simulink model "Sixphase_PMSM_VSD_Robj"  (R2023b)
settings: Solver=ode23t  StartTime=0.0  StopTime=0.5  RelTol=1e-4  EnableMultiTasking=on
InitFcn:
  | Ts=1e-6;
undefined symbols (not defined in the file): DiscIntNeverNeededParam
libraries: spsVoltageMeasurementLib x4, powerlib_extras x3, spsUniversalBridgeLib x2, spsDCVoltageSourceLib x1, spspowerguiLib x1
settings Model: Creator=y  LastModifiedBy=Guoguo
settings SolverCC: AlgebraicLoopSolver=TrustRegion
settings DataIOCC: LimitDataPoints=on  SaveFormat=Array  SignalLoggingSaveFormat=ModelDataLogs  ReturnWorkspaceOutputs=off
settings OptimizationCC: ExpressionDepthLimit=2147483647  InitFltsAndDblsToZero=on  LifeSpan=inf
settings DebuggingCC: SaveWithParameterizedLinksMsg=none  UnderspecifiedInitializationDetection=Classic  MergeDetectMultiDrivingBlocksExec=none  SignalResolutionControl=TryResolveAllWithWarning  SolverPrmCheckMsg=warning  MultiTaskDSMMsg=warning  MultiTaskCondExecSysMsg=none  FcnCallInpInsideContextMsg=warning  UnconnectedInputMsg=warning  UnconnectedOutputMsg=warning  UnconnectedLineMsg=warning  StateNameClashWarn=warning  SFUnexpectedBacktrackingDiag=warning  SFNoUnconditionalDefaultTransitionDiag=warning  SFExecutionAtInitializationDiag=none  ArithmeticOperatorsInVariantConditions=warning
settings HardwareCC: ProdBitPerPointer=32  ProdBitPerSizeT=32  ProdBitPerPtrDiffT=32  ProdLargestAtomicFloat=None  ProdIntDivRoundTo=Undefined  ProdEndianess=Unspecified  ProdWordSize=32  ProdHWDeviceType=32-bit Generic
settings ModelReferenceCC: EnableRefExpFcnMdlSchedulingChecks=on  PropagateSignalLabelsOutOfModel=off
settings SFSimCC: SimUseLocalCustomCode=off  CustomCodeUndefinedFunction=UseInterfaceOnly
settings RTWCC: RTWUseLocalCustomCode=off  DLArmComputeVersion=19.05
settings CodeAppCC: StateflowObjectComments=on
settings GRTTargetCC: TargetFcnLib=ansi_tfl_tmw.mat  TargetLangStandard=C89/C90 (ANSI)  CombineOutputUpdateFcns=off  GRTInterface=on
settings ConfigComp: CovMetricSettings=dw  CovSaveCumulativeToWorkspaceVar=on  CovSaveSingleToWorkspaceVar=on  CovExternalEMLEnable=off  CovSFcnEnable=off
settings SimscapeCC: SimscapeNormalizeSystem=off

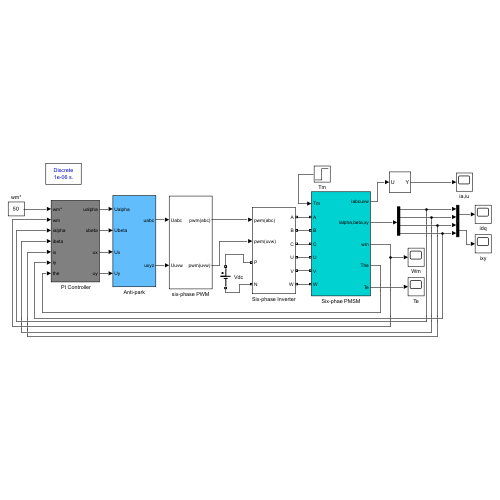
[thumbnail: Simulink's stored preview of the top-level diagram]
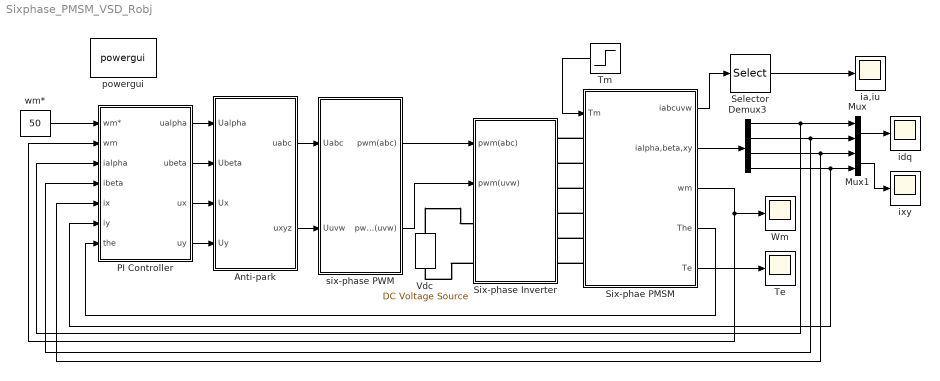
== system Sixphase_PMSM_VSD_Robj ==
  " PI Controller" : Subsystem
  Anti-park : Subsystem
  Demux3 : Demux
  Mux : Mux  Inputs=2
  Mux1 : Mux  Inputs=2
  Selector : Selector  InputPortWidth=6  IndexOptions=Index vector (dialog)  Indices=[1 4]  OutputSizes=1
  Six-phae PMSM : Subsystem  mask{R=1.4, Ld=0.008, Lq=0.008, Lz=0.0017, Flux=0.68, J=0.015, F=0, p=3}
      mask prompts: R "R(ohm)"; Ld "Ld(H)"; Lq "Lq(H)"; Lz "Lz(H)"; Flux "Flux(Wb)"; J "J(kg.m^2)"; F "F(N.m.s)"
  Six-phase Inverter : Subsystem
  Te : Scope
  Tm : Step  Time=0.2  After=50  SampleTime=0
  Vdc : spsDCVoltageSourceLib/DC Voltage Source  Amplitude=400  Measurements=None
  Wm : Scope
  ia,iu : Scope
  idq : Scope
  ixy : Scope
  powergui : spspowerguiLib/powergui  Priority=1  SimulationMode=Discrete  SampleTime=1e-6  frequency=60  Iterations=50  frequencyindice=0  Pbase=100e6  ErrMax=1e-4  UnitsV=kV  UnitsW=MW  buscounter=0  FunctionMessages=off  echomessages=off  EnableUseOfTLC=off  CurrentSourceSwitches=on  DisableSnubberDevices=off  DisableRonSwitches=off  DisableVfSwitches=off  DisplayEquations=off  AutomaticDiscreteSolvers=off  SolverType=Tustin/Backward Euler (TBE)  Interpol=off  ExternalGateDelay=off  methode=off  Ts=100  x0status=blocks  SPID=off  SwTol=0  HookPort=off  NonlinearTolerance=1e-4  nMaxIteration=100  ContinueOnMaxIteration=off  RestoreLinks=warning  ResistiveCurrentMeasurement=off  Frange=[0:2:500]  Ylog=off  Xlog=on  ShowGrid=off  save=off  variable=ZData  structure=iau  ZoomFFT=off  StartTime=0.4  cycles=2  DisplayStyle=1  fundamental=25  FreqAxis=off  MaxFrequency=1000  frequencyindicesteady=1  RmsSteady=1  display=off
  six-phase PWM : Subsystem
  wm* : Constant  Value=50
  wires:
  Six-phae PMSM/4(The) -> " PI Controller"/7(the)
  wm*/1 -> " PI Controller"/1(wm*)
  Six-phae PMSM/2(ialpha,beta,xy) -> Demux3/1
  Six-phae PMSM/5(Te) -> Te/1
  " PI Controller"/1(ualpha) -> Anti-park/1(Ualpha)
  " PI Controller"/2(ubeta) -> Anti-park/2(Ubeta)
  " PI Controller"/3(ux) -> Anti-park/3(Ux)
  " PI Controller"/4(uy) -> Anti-park/4(Uy)
  Demux3/1 -> Mux/1, " PI Controller"/3(ialpha)
  Demux3/2 -> Mux/2, " PI Controller"/4(ibeta)
  Demux3/3 -> " PI Controller"/5(ix), Mux1/1
  Demux3/4 -> " PI Controller"/6(iy), Mux1/2
  Tm/1 -> Six-phae PMSM/1(Tm)
  Anti-park/1(uabc) -> six-phase PWM/1(Uabc)
  Anti-park/2(uxyz) -> six-phase PWM/2(Uuvw)
  six-phase PWM/1(pwm(abc)) -> Six-phase Inverter/1(pwm(abc))
  six-phase PWM/2(pwm(uvw)) -> Six-phase Inverter/2(pwm(uvw))
  Six-phae PMSM/3(wm) -> Wm/1, " PI Controller"/2(wm)
  Mux/1 -> idq/1
  Mux1/1 -> ixy/1
  Selector/1 -> ia,iu/1
  Six-phae PMSM/1(iabcuvw) -> Selector/1
  connections:
  Six-phae PMSM/LConn1 -- Six-phase Inverter/RConn1
  Six-phae PMSM/LConn2 -- Six-phase Inverter/RConn2
  Six-phae PMSM/LConn3 -- Six-phase Inverter/RConn3
  Six-phae PMSM/LConn4 -- Six-phase Inverter/RConn4
  Six-phae PMSM/LConn5 -- Six-phase Inverter/RConn5
  Six-phae PMSM/LConn6 -- Six-phase Inverter/RConn6
  Vdc/RConn1 -- Six-phase Inverter/LConn1
  Six-phase Inverter/LConn2 -- Vdc/LConn1

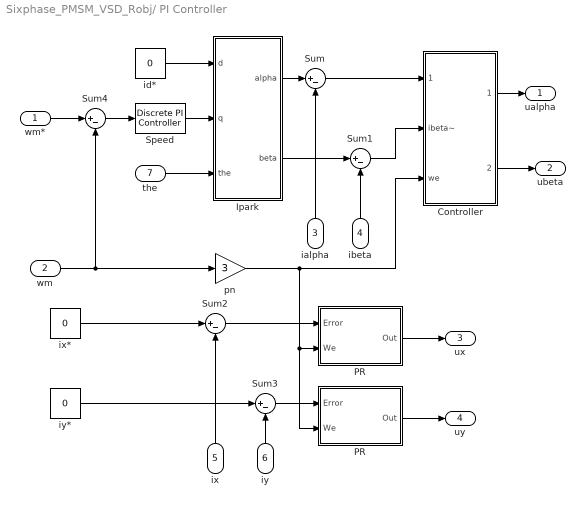
== system Sixphase_PMSM_VSD_Robj/ PI Controller ==
  wm* : Inport
  wm : Inport  Port=2
  ialpha : Inport  Port=3
  ibeta : Inport  Port=4
  ix : Inport  Port=5
  iy : Inport  Port=6
  the : Inport  Port=7
  Controller : Subsystem  AncestorBlock=|  DialogController=POWERSYS.PowerSysDialog  mask(Discrete PI Controller){Kp=0.008*1200, Ki=1.4*1200, Par_Limits=[100 -100], Init=0, Ts=Ts}
      | powerlib_extras/Discrete 
      | Control Blocks/Discrete
      | PI Controller
      mask prompts: Kp "Proportional gain (Kp):"; Ki "Integral gain (Ki):"; Par_Limits "Output limits: [ Upper   Lower ]"; Init "Output initial value:"; Ts "Sample time:"
      mask help: This block implements a discrete PI controller.
      mask init:
      | UpperLimit=Par_Limits(1);
      | LowerLimit=Par_Limits(2);
      | power_initmask();
      mask Help: This block is part of a subset of blocks in the Extras library that does not have documentation associated with it, other than the block mask description.
  Ipark : Subsystem
  PR : Subsystem  AncestorBlock=|  DialogController=POWERSYS.PowerSysDialog  mask(Discrete PI Controller){Kp=0.0017*1200, wc=20, ki=100, Par_Limits=[300/sqrt(3) -300/sqrt(3)], Init=0, Ts=Ts}
      | powerlib_extras/Discrete 
      | Control Blocks/Discrete
      | PI Controller
      mask prompts: Kp "Proportional gain (Kp):"; wc "Cut-off frequency(wc)"; ki "PR integral gain (ki)"; Par_Limits "Output limits: [ Upper   Lower ]"; Init "Output initial value:"; Ts "Sample time:"
      mask help: This block implements a discrete PI controller.
      mask init:
      | UpperLimit=Par_Limits(1);
      | LowerLimit=Par_Limits(2);
      | power_initmask();
      mask Help: This block is part of a subset of blocks in the Extras library that does not have documentation associated with it, other than the block mask description.
  "PR " : Subsystem  AncestorBlock=|  DialogController=POWERSYS.PowerSysDialog  mask(Discrete PI Controller){Kp=0.0017*1200, wc=20, ki=100, Par_Limits=[300/sqrt(3) -300/sqrt(3)], Init=0, Ts=Ts}
      | powerlib_extras/Discrete 
      | Control Blocks/Discrete
      | PI Controller
      mask prompts: Kp "Proportional gain (Kp):"; wc "Cut-off frequency(wc)"; ki "PR integral gain (ki)"; Par_Limits "Output limits: [ Upper   Lower ]"; Init "Output initial value:"; Ts "Sample time:"
      mask help: This block implements a discrete PI controller.
      mask init:
      | UpperLimit=Par_Limits(1);
      | LowerLimit=Par_Limits(2);
      | power_initmask();
      mask Help: This block is part of a subset of blocks in the Extras library that does not have documentation associated with it, other than the block mask description.
  Speed : powerlib_extras/Discrete  Control Blocks/Discrete PI Controller  Kp=1  Ki=80  Par_Limits=[25 -25]  Init=0  Ts=Ts
  Sum{,1..4} (5 alike) : Sum  Inputs=|+-
  id* : Constant  Value=0
  ix* : Constant  Value=0
  iy* : Constant  Value=0
  pn : Gain  Gain=3
  ualpha : Outport
  ubeta : Outport  Port=2
  ux : Outport  Port=3
  uy : Outport  Port=4
  wires:
  Sum3/1 -> "PR "/1(Error)
  Sum2/1 -> PR/1(Error)
  Sum1/1 -> Controller/2(ibeta~)
  Sum/1 -> Controller/1(ialpha~)
  Sum4/1 -> Speed/1
  ix/1 -> Sum2/2
  iy/1 -> Sum3/2
  Controller/1(Valpha*) -> ualpha/1
  Controller/2(Vbeta*) -> ubeta/1
  ix*/1 -> Sum2/1
  iy*/1 -> Sum3/1
  PR/1(Out) -> ux/1
  "PR "/1(Out) -> uy/1
  Ipark/1(alpha) -> Sum/1
  id*/1 -> Ipark/1(d)
  Speed/1 -> Ipark/2(q)
  Ipark/2(beta) -> Sum1/1
  the/1 -> Ipark/3(the)
  ialpha/1 -> Sum/2
  ibeta/1 -> Sum1/2
  wm/1 -> pn/1, Sum4/2
  wm*/1 -> Sum4/1
  pn/1 -> "PR "/2(We), PR/2(We), Controller/3(we)

== system Sixphase_PMSM_VSD_Robj/Anti-park ==
  Ualpha : Inport
  Ubeta : Inport  Port=2
  Ux : Inport  Port=3
  Uy : Inport  Port=4
  Demux : Demux  Outputs=2
  Gain : Gain  Gain=1/200
  IClarke-6 : Subsystem
  uabc : Outport
  uxyz : Outport  Port=2
  wires:
  IClarke-6/1(ABCUVW) -> Gain/1
  Ualpha/1 -> IClarke-6/1(alpha)
  Ubeta/1 -> IClarke-6/2(beta)
  Ux/1 -> IClarke-6/3(x)
  Uy/1 -> IClarke-6/4(y)
  Gain/1 -> Demux/1
  Demux/1 -> uabc/1
  Demux/2 -> uxyz/1

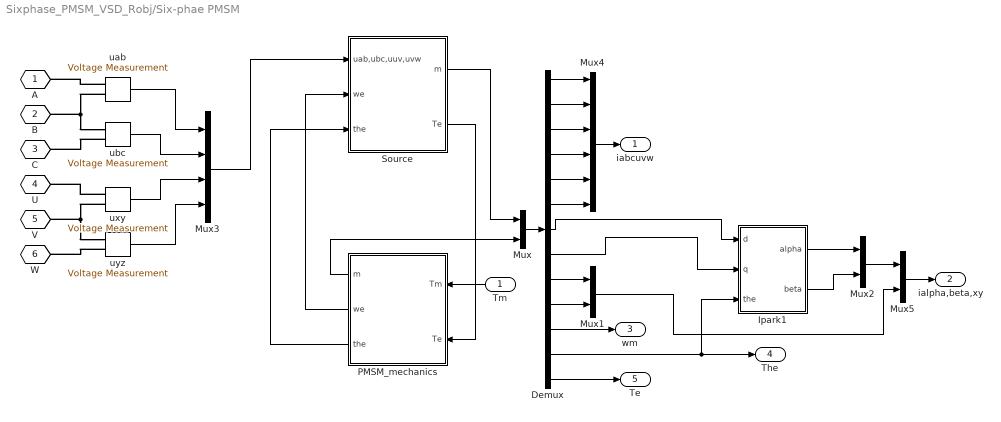
== system Sixphase_PMSM_VSD_Robj/Six-phae PMSM ==
  Tm : Inport
  Demux : Demux  Outputs=13
  Ipark1 : Subsystem
  Mux{,1..2,5} (4 alike) : Mux  Inputs=2
  Mux3 : Mux
  Mux4 : Mux  Inputs=6
  PMSM_mechanics : Subsystem
  Source : Subsystem
  uab : spsVoltageMeasurementLib/Voltage Measurement  PhasorSimulation=off  OutputType=Complex  PSBequivalent=0
  ubc : spsVoltageMeasurementLib/Voltage Measurement  PhasorSimulation=off  OutputType=Complex  PSBequivalent=0
  uxy : spsVoltageMeasurementLib/Voltage Measurement  PhasorSimulation=off  OutputType=Complex  PSBequivalent=0
  uyz : spsVoltageMeasurementLib/Voltage Measurement  PhasorSimulation=off  OutputType=Complex  PSBequivalent=0
  A : PMIOPort  Tag=PMCPort  Side=Left
  B : PMIOPort  Tag=PMCPort  Port=2  Side=Left
  C : PMIOPort  Tag=PMCPort  Port=3  Side=Left
  U : PMIOPort  Tag=PMCPort  Port=4  Side=Left
  V : PMIOPort  Tag=PMCPort  Port=5  Side=Left
  W : PMIOPort  Tag=PMCPort  Port=6  Side=Left
  iabcuvw : Outport
  ialpha,beta,xy : Outport  Port=2
  wm : Outport  Port=3
  The : Outport  Port=4
  Te : Outport  Port=5
  wires:
  Tm/1 -> PMSM_mechanics/1(Tm)
  Source/2(Te) -> PMSM_mechanics/2(Te)
  PMSM_mechanics/2(we) -> Source/2(we)
  PMSM_mechanics/3(the) -> Source/3(the)
  PMSM_mechanics/1(m) -> Mux/2
  Source/1(m) -> Mux/1
  Mux3/1 -> Source/1(uab,ubc,uuv,uvw)
  Mux/1 -> Demux/1
  Mux4/1 -> iabcuvw/1
  Mux5/1 -> ialpha,beta,xy/1
  Demux/12 -> Ipark1/3(the), The/1
  Demux/13 -> Te/1
  uab/1 -> Mux3/1
  ubc/1 -> Mux3/2
  uxy/1 -> Mux3/3
  uyz/1 -> Mux3/4
  Demux/5 -> Mux4/5
  Demux/2 -> Mux4/2
  Demux/3 -> Mux4/3
  Demux/6 -> Mux4/6
  Demux/4 -> Mux4/4
  Demux/1 -> Mux4/1
  Demux/7 -> Ipark1/1(d)
  Demux/8 -> Ipark1/2(q)
  Demux/9 -> Mux1/1
  Demux/10 -> Mux1/2
  Demux/11 -> wm/1
  Ipark1/1(alpha) -> Mux2/1
  Ipark1/2(beta) -> Mux2/2
  Mux2/1 -> Mux5/1
  Mux1/1 -> Mux5/2
  connections:
  uab/LConn1 -- A/RConn1
  uab/LConn2 -- B/RConn1 -- ubc/LConn1
  ubc/LConn2 -- C/RConn1
  uxy/LConn1 -- U/RConn1
  uxy/LConn2 -- V/RConn1 -- uyz/LConn1
  uyz/LConn2 -- W/RConn1

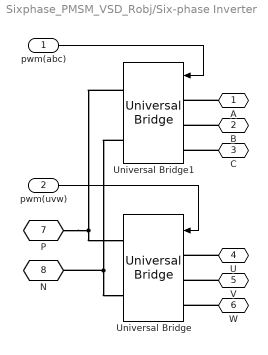
== system Sixphase_PMSM_VSD_Robj/Six-phase Inverter ==
  pwm(abc) : Inport
  pwm(uvw) : Inport  Port=2
  Universal Bridge : spsUniversalBridgeLib/Universal Bridge  Arms=3  SnubberResistance=1e5  SnubberCapacitance=inf  Device=IGBT / Diodes  Ron=1e-3  Lon=0  ForwardVoltages="[  0  0  ]"  ForwardVoltage=0  GTOparameters=[ 10e-6 , 20e-6 ]  IGBTparameters=[ 1e-6 , 2e-6 ]  Measurements=None  Measurements_2=None  converterType=Rectifier
  Universal Bridge1 : spsUniversalBridgeLib/Universal Bridge  Arms=3  SnubberResistance=1e5  SnubberCapacitance=inf  Device=IGBT / Diodes  Ron=1e-3  Lon=0  ForwardVoltages="[  0  0  ]"  ForwardVoltage=0  GTOparameters=[ 10e-6 , 20e-6 ]  IGBTparameters=[ 1e-6 , 2e-6 ]  Measurements=None  Measurements_2=None  converterType=Rectifier
  A : PMIOPort  Side=Right
  B : PMIOPort  Port=2  Side=Right
  C : PMIOPort  Port=3  Side=Right
  U : PMIOPort  Port=4  Side=Right
  V : PMIOPort  Port=5  Side=Right
  W : PMIOPort  Port=6  Side=Right
  P : PMIOPort  Port=7  Side=Left
  N : PMIOPort  Port=8  Side=Left
  wires:
  pwm(abc)/1 -> Universal Bridge1/1
  pwm(uvw)/1 -> Universal Bridge/1
  connections:
  A/RConn1 -- Universal Bridge1/LConn1
  C/RConn1 -- Universal Bridge1/LConn3
  W/RConn1 -- Universal Bridge/LConn3
  B/RConn1 -- Universal Bridge1/LConn2
  U/RConn1 -- Universal Bridge/LConn1
  V/RConn1 -- Universal Bridge/LConn2
  Universal Bridge1/RConn1 -- P/RConn1 -- Universal Bridge/RConn1
  Universal Bridge1/RConn2 -- N/RConn1 -- Universal Bridge/RConn2

== system Sixphase_PMSM_VSD_Robj/six-phase PWM ==
  Uabc : Inport
  Uuvw : Inport  Port=2
  Discrete PWM Generator : powerlib_extras/Discrete  Control Blocks/Discrete PWM Generator  GeneratorMode="3-arm  bridge (6 pulses)"  Fc=10000  Ts=1e-6  Internal=off  mIndex=0.4  Freq=60  Phase=0
  Discrete PWM Generator1 : powerlib_extras/Discrete  Control Blocks/Discrete PWM Generator  GeneratorMode="3-arm  bridge (6 pulses)"  Fc=10000  Ts=1e-6  Internal=off  mIndex=0.4  Freq=60  Phase=0
  pwm(abc) : Outport
  pwm(uvw) : Outport  Port=2
  wires:
  Uabc/1 -> Discrete PWM Generator/1
  Discrete PWM Generator1/1 -> pwm(uvw)/1
  Uuvw/1 -> Discrete PWM Generator1/1
  Discrete PWM Generator/1 -> pwm(abc)/1

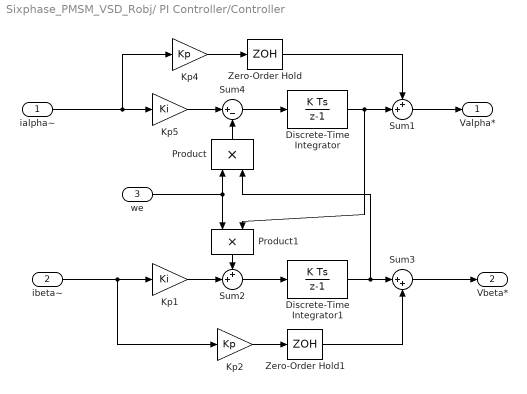
== system Sixphase_PMSM_VSD_Robj/ PI Controller/Controller ==
  ialpha~ : Inport  SampleTime=Ts
  ibeta~ : Inport  Port=2  SampleTime=Ts
  we : Inport  Port=3  SampleTime=Ts
  Discrete-Time Integrator : DiscreteIntegrator  InitialCondition=Init  SampleTime=Ts  UpperSaturationLimit=UpperLimit  LowerSaturationLimit=LowerLimit  ICPrevOutput=DiscIntNeverNeededParam  ICPrevScaledInput=DiscIntNeverNeededParam
  Discrete-Time Integrator1 : DiscreteIntegrator  InitialCondition=Init  SampleTime=Ts  UpperSaturationLimit=UpperLimit  LowerSaturationLimit=LowerLimit  ICPrevOutput=DiscIntNeverNeededParam  ICPrevScaledInput=DiscIntNeverNeededParam
  Kp1 : Gain  Gain=Ki  SaturateOnIntegerOverflow=on  SampleTime=Ts  OutDataTypeStr=Inherit: Same as input  ParamDataTypeStr=Inherit: Same as input
  Kp2 : Gain  Gain=Kp  SaturateOnIntegerOverflow=on  SampleTime=Ts  OutDataTypeStr=Inherit: Same as input  ParamDataTypeStr=Inherit: Same as input
  Kp4 : Gain  Gain=Kp  SaturateOnIntegerOverflow=on  SampleTime=Ts  OutDataTypeStr=Inherit: Same as input  ParamDataTypeStr=Inherit: Same as input
  Kp5 : Gain  Gain=Ki  SaturateOnIntegerOverflow=on  SampleTime=Ts  OutDataTypeStr=Inherit: Same as input  ParamDataTypeStr=Inherit: Same as input
  Product : Product
  Product1 : Product
  Sum1 : Sum  Inputs=++|
  Sum2 : Sum  Inputs=++|
  Sum3 : Sum  Inputs=|++
  Sum4 : Sum  Inputs=|+-
  Zero-Order Hold : ZeroOrderHold  SampleTime=Ts
  Zero-Order Hold1 : ZeroOrderHold  SampleTime=Ts
  Valpha* : Outport  SampleTime=Ts  InitialOutput=0
  Vbeta* : Outport  Port=2  SampleTime=Ts  InitialOutput=0
  wires:
  ialpha~/1 -> Kp4/1, Kp5/1
  Kp4/1 -> Zero-Order Hold/1
  Sum1/1 -> Valpha*/1
  Zero-Order Hold/1 -> Sum1/1
  Kp5/1 -> Sum4/1
  Sum4/1 -> Discrete-Time Integrator/1
  Product/1 -> Sum4/2
  we/1 -> Product1/1, Product/1
  Sum2/1 -> Discrete-Time Integrator1/1
  Kp1/1 -> Sum2/2
  Kp2/1 -> Zero-Order Hold1/1
  ibeta~/1 -> Kp2/1, Kp1/1
  Zero-Order Hold1/1 -> Sum3/2
  Discrete-Time Integrator1/1 -> Product/2, Sum3/1
  Product1/1 -> Sum2/1
  Discrete-Time Integrator/1 -> Product1/2, Sum1/2
  Sum3/1 -> Vbeta*/1

== system Sixphase_PMSM_VSD_Robj/ PI Controller/Ipark ==
  d : Inport
  q : Inport  Port=2
  the : Inport  Port=3
  Fcn : Fcn  Expr=u[1]*u[4]-u[2]*u[3]
  Fcn1 : Fcn  Expr=u[1]*u[3]+u[2]*u[4]
  Mux : Mux
  cos : Trigonometry  Operator=cos
  sin : Trigonometry
  alpha : Outport
  beta : Outport  Port=2
  wires:
  d/1 -> Mux/1
  q/1 -> Mux/2
  Mux/1 -> Fcn1/1, Fcn/1
  sin/1 -> Mux/3
  cos/1 -> Mux/4
  the/1 -> sin/1, cos/1
  Fcn/1 -> alpha/1
  Fcn1/1 -> beta/1

== system Sixphase_PMSM_VSD_Robj/ PI Controller/PR ==
  note: Discrete PID Controller
  note: Pierre Giroux, Gilbert Sybille
      | Power System Simulation Laboratory
      | IREQ, Hydro-Quebc
  Error : Inport  SampleTime=Ts
  We : Inport  Port=2  SampleTime=Ts
  Kp4 : Gain  Gain=Kp  SaturateOnIntegerOverflow=on  SampleTime=Ts  OutDataTypeStr=Inherit: Same as input  ParamDataTypeStr=Inherit: Same as input
  PR : Subsystem
  Sum6 : Sum  InputSameDT=on  SaturateOnIntegerOverflow=on  SampleTime=Ts  OutDataTypeStr=Inherit: Same as first input
  Zero-Order Hold : ZeroOrderHold  SampleTime=Ts
  Out : Outport  SampleTime=Ts  InitialOutput=0
  wires:
  PR/1(Out) -> Sum6/2
  We/1 -> PR/2(we)
  Zero-Order Hold/1 -> Sum6/1
  Sum6/1 -> Out/1
  Kp4/1 -> Zero-Order Hold/1
  Error/1 -> PR/1(error), Kp4/1

== system Sixphase_PMSM_VSD_Robj/ PI Controller/PR  ==
  note: Pierre Giroux, Gilbert Sybille
      | Power System Simulation Laboratory
      | IREQ, Hydro-Quebc
  note: Discrete PID Controller
  Error : Inport  SampleTime=Ts
  We : Inport  Port=2  SampleTime=Ts
  Kp4 : Gain  Gain=Kp  SaturateOnIntegerOverflow=on  SampleTime=Ts  OutDataTypeStr=Inherit: Same as input  ParamDataTypeStr=Inherit: Same as input
  PR : Subsystem
  Sum6 : Sum  InputSameDT=on  SaturateOnIntegerOverflow=on  SampleTime=Ts  OutDataTypeStr=Inherit: Same as first input
  Zero-Order Hold : ZeroOrderHold  SampleTime=Ts
  Out : Outport  SampleTime=Ts  InitialOutput=0
  wires:
  Error/1 -> Kp4/1, PR/1(error)
  Kp4/1 -> Zero-Order Hold/1
  Sum6/1 -> Out/1
  Zero-Order Hold/1 -> Sum6/1
  We/1 -> PR/2(we)
  PR/1(Out) -> Sum6/2

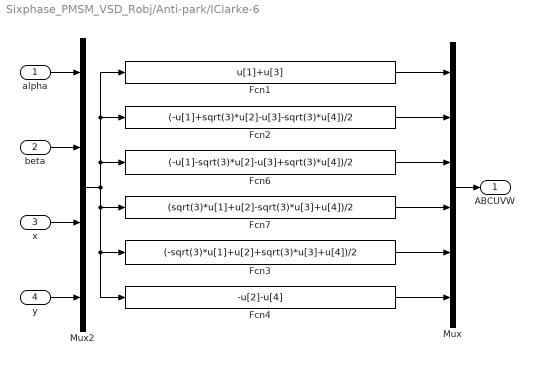
== system Sixphase_PMSM_VSD_Robj/Anti-park/IClarke-6 ==
  alpha : Inport
  beta : Inport  Port=2
  x : Inport  Port=3
  y : Inport  Port=4
  Fcn1 : Fcn  Expr=u[1]+u[3]
  Fcn2 : Fcn  Expr=(-u[1]+sqrt(3)*u[2]-u[3]-sqrt(3)*u[4])/2
  Fcn3 : Fcn  Expr=(-sqrt(3)*u[1]+u[2]+sqrt(3)*u[3]+u[4])/2
  Fcn4 : Fcn  Expr=-u[2]-u[4]
  Fcn6 : Fcn  Expr=(-u[1]-sqrt(3)*u[2]-u[3]+sqrt(3)*u[4])/2
  Fcn7 : Fcn  Expr=(sqrt(3)*u[1]+u[2]-sqrt(3)*u[3]+u[4])/2
  Mux : Mux  Inputs=6
  Mux2 : Mux
  ABCUVW : Outport
  wires:
  alpha/1 -> Mux2/1
  beta/1 -> Mux2/2
  x/1 -> Mux2/3
  y/1 -> Mux2/4
  Mux2/1 -> Fcn7/1, Fcn3/1, Fcn4/1, Fcn1/1, Fcn2/1, Fcn6/1
  Fcn1/1 -> Mux/1
  Fcn2/1 -> Mux/2
  Fcn6/1 -> Mux/3
  Fcn7/1 -> Mux/4
  Fcn3/1 -> Mux/5
  Fcn4/1 -> Mux/6
  Mux/1 -> ABCUVW/1

== system Sixphase_PMSM_VSD_Robj/Six-phae PMSM/Ipark1 ==
  d : Inport
  q : Inport  Port=2
  the : Inport  Port=3
  Fcn : Fcn  Expr=u[1]*u[4]-u[2]*u[3]
  Fcn1 : Fcn  Expr=u[1]*u[3]+u[2]*u[4]
  Mux : Mux
  cos : Trigonometry  Operator=cos
  sin : Trigonometry
  alpha : Outport
  beta : Outport  Port=2
  wires:
  Fcn1/1 -> beta/1
  Fcn/1 -> alpha/1
  the/1 -> cos/1, sin/1
  cos/1 -> Mux/4
  sin/1 -> Mux/3
  Mux/1 -> Fcn/1, Fcn1/1
  q/1 -> Mux/2
  d/1 -> Mux/1

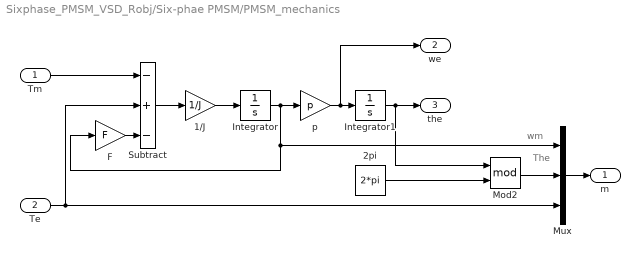
== system Sixphase_PMSM_VSD_Robj/Six-phae PMSM/PMSM_mechanics ==
  note: The
  note: wm
  Tm : Inport
  Te : Inport  Port=2
  1/J : Gain  Gain=1/J
  2pi : Constant  Value=2*pi
  F : Gain  Gain=F
  Integrator : Integrator
  Integrator1 : Integrator
  Mod2 : Math  Operator=mod  SignedPower=on
  Mux : Mux  Inputs=3
  Subtract : Sum  Inputs=-+-
  p : Gain  Gain=p
  m : Outport
  we : Outport  Port=2
  the : Outport  Port=3
  wires:
  Tm/1 -> Subtract/1
  Te/1 -> Subtract/2, Mux/3
  Subtract/1 -> 1/J/1
  1/J/1 -> Integrator/1
  Integrator/1 -> p/1, F/1, Mux/1
  F/1 -> Subtract/3
  p/1 -> Integrator1/1, we/1
  Integrator1/1 -> the/1, Mod2/1
  Mux/1 -> m/1
  Mod2/1 -> Mux/2
  2pi/1 -> Mod2/2

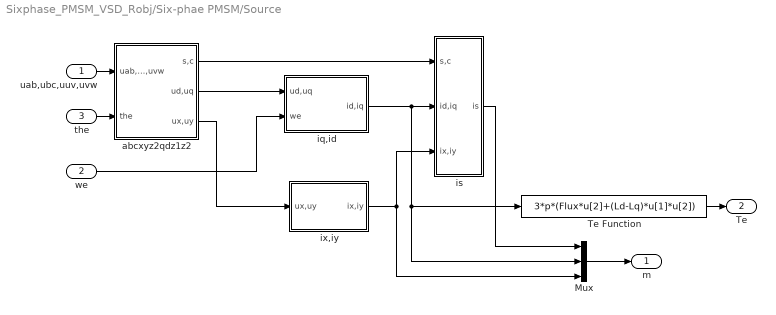
== system Sixphase_PMSM_VSD_Robj/Six-phae PMSM/Source ==
  uab,ubc,uuv,uvw : Inport
  we : Inport  Port=2
  the : Inport  Port=3
  Mux : Mux  Inputs=3
  Te Function : Fcn  Expr=3*p*(Flux*u[2]+(Ld-Lq)*u[1]*u[2])
  abcxyz2qdz1z2 : Subsystem
  iq,id : Subsystem
  is : Subsystem
  ix,iy : Subsystem
  m : Outport
  Te : Outport  Port=2
  wires:
  uab,ubc,uuv,uvw/1 -> abcxyz2qdz1z2/1(uab,ubc,uuv,uvw)
  the/1 -> abcxyz2qdz1z2/2(the)
  abcxyz2qdz1z2/2(ud,uq) -> iq,id/1(ud,uq)
  we/1 -> iq,id/2(we)
  abcxyz2qdz1z2/1(s,c) -> is/1(s,c)
  iq,id/1(id,iq) -> is/2(id,iq), Mux/2, Te Function/1
  Te Function/1 -> Te/1
  abcxyz2qdz1z2/3(ux,uy) -> ix,iy/1(ux,uy)
  ix,iy/1(ix,iy) -> is/3(ix,iy), Mux/3
  Mux/1 -> m/1
  is/1(is) -> Mux/1

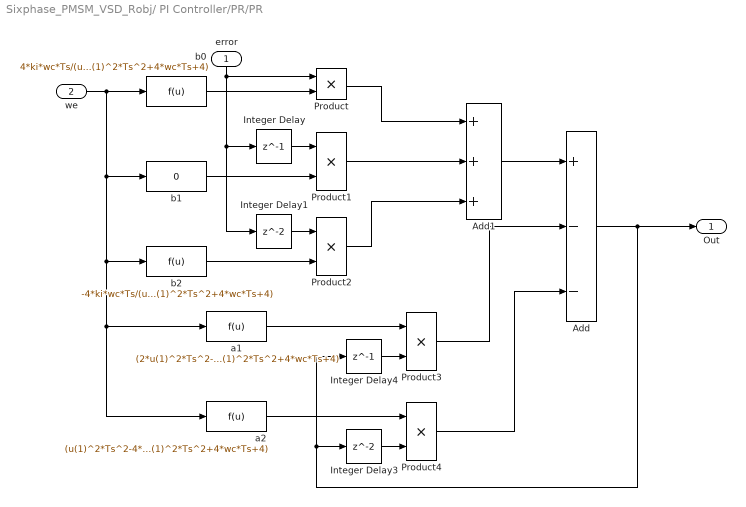
== system Sixphase_PMSM_VSD_Robj/ PI Controller/PR/PR ==
  error : Inport
  we : Inport  Port=2
  Add : Sum  Inputs=+--
  Add1 : Sum  Inputs=+++
  Integer Delay : Delay  DelayLength=1  SampleTime=Ts
  Integer Delay1 : Delay  SampleTime=Ts
  Integer Delay3 : Delay
  Integer Delay4 : Delay  DelayLength=1  SampleTime=Ts
  Product{,1..4} (5 alike) : Product  RndMeth=Zero
  a1 : Fcn  Expr=(2*u(1)^2*Ts^2-8)/(u(1)^2*Ts^2+4*wc*Ts+4)  SampleTime=Ts
  a2 : Fcn  Expr=(u(1)^2*Ts^2-4*wc*Ts+4)/(u(1)^2*Ts^2+4*wc*Ts+4)  SampleTime=Ts
  b0 : Fcn  Expr=4*ki*wc*Ts/(u(1)^2*Ts^2+4*wc*Ts+4)
  b1 : Fcn  Expr=0
  b2 : Fcn  Expr=-4*ki*wc*Ts/(u(1)^2*Ts^2+4*wc*Ts+4)
  Out : Outport
  wires:
  we/1 -> b0/1, b1/1, b2/1, a1/1, a2/1
  b0/1 -> Product/2
  b1/1 -> Product1/2
  Integer Delay/1 -> Product1/1
  Integer Delay1/1 -> Product2/1
  b2/1 -> Product2/2
  Product/1 -> Add1/1
  Product1/1 -> Add1/2
  Product2/1 -> Add1/3
  Add/1 -> Out/1, Integer Delay4/1, Integer Delay3/1
  a1/1 -> Product3/1
  a2/1 -> Product4/1
  Integer Delay3/1 -> Product4/2
  Integer Delay4/1 -> Product3/2
  Add1/1 -> Add/1
  Product3/1 -> Add/2
  Product4/1 -> Add/3
  error/1 -> Product/1, Integer Delay/1, Integer Delay1/1

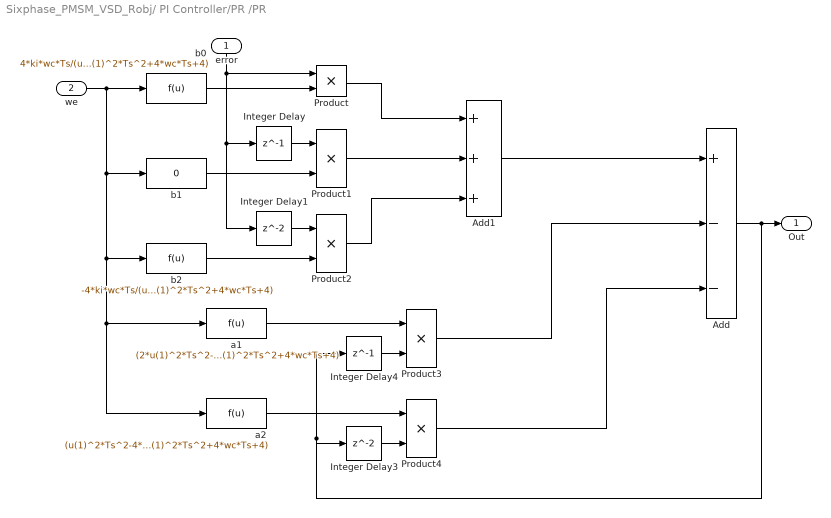
== system Sixphase_PMSM_VSD_Robj/ PI Controller/PR /PR ==
  error : Inport
  we : Inport  Port=2
  Add : Sum  Inputs=+--
  Add1 : Sum  Inputs=+++
  Integer Delay : Delay  DelayLength=1  SampleTime=Ts
  Integer Delay1 : Delay  SampleTime=Ts
  Integer Delay3 : Delay
  Integer Delay4 : Delay  DelayLength=1  SampleTime=Ts
  Product{,1..4} (5 alike) : Product  RndMeth=Zero
  a1 : Fcn  Expr=(2*u(1)^2*Ts^2-8)/(u(1)^2*Ts^2+4*wc*Ts+4)  SampleTime=Ts
  a2 : Fcn  Expr=(u(1)^2*Ts^2-4*wc*Ts+4)/(u(1)^2*Ts^2+4*wc*Ts+4)  SampleTime=Ts
  b0 : Fcn  Expr=4*ki*wc*Ts/(u(1)^2*Ts^2+4*wc*Ts+4)
  b1 : Fcn  Expr=0
  b2 : Fcn  Expr=-4*ki*wc*Ts/(u(1)^2*Ts^2+4*wc*Ts+4)
  Out : Outport
  wires:
  error/1 -> Integer Delay1/1, Integer Delay/1, Product/1
  Product4/1 -> Add/3
  Product3/1 -> Add/2
  Add1/1 -> Add/1
  Integer Delay4/1 -> Product3/2
  Integer Delay3/1 -> Product4/2
  a2/1 -> Product4/1
  a1/1 -> Product3/1
  Add/1 -> Out/1, Integer Delay3/1, Integer Delay4/1
  Product2/1 -> Add1/3
  Product1/1 -> Add1/2
  Product/1 -> Add1/1
  b2/1 -> Product2/2
  Integer Delay1/1 -> Product2/1
  Integer Delay/1 -> Product1/1
  b1/1 -> Product1/2
  b0/1 -> Product/2
  we/1 -> a2/1, a1/1, b2/1, b1/1, b0/1

== system Sixphase_PMSM_VSD_Robj/Six-phae PMSM/Source/abcxyz2qdz1z2 ==
  uab,ubc,uuv,uvw : Inport
  the : Inport  Port=2
  Clarke : Subsystem
  Mux2 : Mux  Inputs=2
  PARK : Subsystem
  Trigonometric Function : Trigonometry
  Trigonometric Function1 : Trigonometry  Operator=cos
  s,c : Outport
  ud,uq : Outport  Port=2
  ux,uy : Outport  Port=3
  wires:
  Mux2/1 -> PARK/2(s,c), s,c/1
  the/1 -> Trigonometric Function1/1, Trigonometric Function/1
  PARK/1(ud,uq) -> ud,uq/1
  uab,ubc,uuv,uvw/1 -> Clarke/1(uab,ubc,uuv,uvw)
  Trigonometric Function1/1 -> Mux2/2
  Trigonometric Function/1 -> Mux2/1
  Clarke/1(ualpha,ubeta) -> PARK/1(ualpha,ubeta)
  Clarke/2(ux,uy) -> ux,uy/1

== system Sixphase_PMSM_VSD_Robj/Six-phae PMSM/Source/iq,id ==
  ud,uq : Inport
  we : Inport  Port=2
  Demux : Demux  Outputs=2
  Mux : Mux  Inputs=2
  id : Subsystem
  iq : Subsystem
  id,iq : Outport
  wires:
  ud,uq/1 -> Demux/1
  Mux/1 -> id,iq/1
  Demux/1 -> id/1(ud)
  Demux/2 -> iq/3(uq)
  we/1 -> iq/2(we), id/2(we)
  iq/1(iq) -> id/3(iq), Mux/2
  id/1(id) -> iq/1(id), Mux/1

== system Sixphase_PMSM_VSD_Robj/Six-phae PMSM/Source/is ==
  s,c : Inport
  id,iq : Inport  Port=2
  ix,iy : Inport  Port=3
  IClarke : Subsystem
  IPARK : Subsystem
  is : Outport
  wires:
  s,c/1 -> IPARK/1(s,c)
  id,iq/1 -> IPARK/2(id,iq)
  IPARK/1(ialpha,ibeta) -> IClarke/1(ialpha,ibeta)
  ix,iy/1 -> IClarke/2(ix,iy)
  IClarke/1(iabcuvw) -> is/1

== system Sixphase_PMSM_VSD_Robj/Six-phae PMSM/Source/ix,iy ==
  ux,uy : Inport
  Demux : Demux  Outputs=2
  Mux : Mux  Inputs=2
  ix : Subsystem
  iy : Subsystem
  ix,iy : Outport
  wires:
  Mux/1 -> ix,iy/1
  ux,uy/1 -> Demux/1
  Demux/1 -> ix/1(ux)
  Demux/2 -> iy/1(uy)
  ix/1(ix) -> Mux/1
  iy/1(iy) -> Mux/2

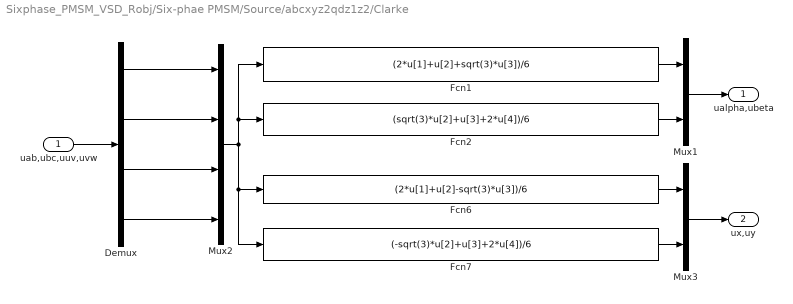
== system Sixphase_PMSM_VSD_Robj/Six-phae PMSM/Source/abcxyz2qdz1z2/Clarke ==
  uab,ubc,uuv,uvw : Inport
  Demux : Demux
  Fcn1 : Fcn  Expr=(2*u[1]+u[2]+sqrt(3)*u[3])/6
  Fcn2 : Fcn  Expr=(sqrt(3)*u[2]+u[3]+2*u[4])/6
  Fcn6 : Fcn  Expr=(2*u[1]+u[2]-sqrt(3)*u[3])/6
  Fcn7 : Fcn  Expr=(-sqrt(3)*u[2]+u[3]+2*u[4])/6
  Mux1 : Mux  Inputs=2
  Mux2 : Mux
  Mux3 : Mux  Inputs=2
  ualpha,ubeta : Outport
  ux,uy : Outport  Port=2
  wires:
  Demux/2 -> Mux2/2
  Demux/3 -> Mux2/3
  Demux/4 -> Mux2/4
  Mux2/1 -> Fcn1/1, Fcn2/1, Fcn6/1, Fcn7/1
  uab,ubc,uuv,uvw/1 -> Demux/1
  Demux/1 -> Mux2/1
  Mux1/1 -> ualpha,ubeta/1
  Fcn1/1 -> Mux1/1
  Fcn2/1 -> Mux1/2
  Fcn6/1 -> Mux3/1
  Fcn7/1 -> Mux3/2
  Mux3/1 -> ux,uy/1

== system Sixphase_PMSM_VSD_Robj/Six-phae PMSM/Source/abcxyz2qdz1z2/PARK ==
  ualpha,ubeta : Inport
  s,c : Inport  Port=2
  Demux : Demux  Outputs=2
  Demux1 : Demux  Outputs=2
  Fcn : Fcn  Expr=u[1]*u[4]+u[2]*u[3]
  Fcn1 : Fcn  Expr=-u[1]*u[3]+u[2]*u[4]
  Mux : Mux
  Mux1 : Mux  Inputs=2
  ud,uq : Outport
  wires:
  Mux/1 -> Fcn/1, Fcn1/1
  s,c/1 -> Demux/1
  ualpha,ubeta/1 -> Demux1/1
  Demux1/1 -> Mux/1
  Demux1/2 -> Mux/2
  Demux/1 -> Mux/3
  Demux/2 -> Mux/4
  Fcn/1 -> Mux1/1
  Fcn1/1 -> Mux1/2
  Mux1/1 -> ud,uq/1

== system Sixphase_PMSM_VSD_Robj/Six-phae PMSM/Source/iq,id/id ==
  ud : Inport
  we : Inport  Port=2
  iq : Inport  Port=3
  1/Ld : Gain  Gain=1/Ld
  Lq/Ld : Gain  Gain=Lq/Ld
  Product : Product  RndMeth=Zero
  R/Ld : Gain  Gain=R/Ld
  Subtract : Sum  Inputs=-++
  d/dt(id) : Integrator
  id : Outport
  wires:
  d/dt(id)/1 -> id/1, R/Ld/1
  Subtract/1 -> d/dt(id)/1
  R/Ld/1 -> Subtract/1
  1/Ld/1 -> Subtract/2
  Lq/Ld/1 -> Subtract/3
  Product/1 -> Lq/Ld/1
  iq/1 -> Product/2
  we/1 -> Product/1
  ud/1 -> 1/Ld/1

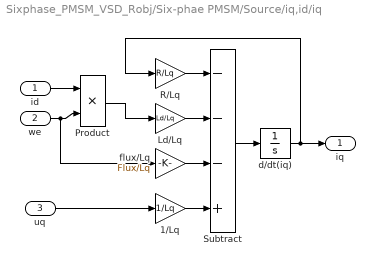
== system Sixphase_PMSM_VSD_Robj/Six-phae PMSM/Source/iq,id/iq ==
  id : Inport
  we : Inport  Port=2
  uq : Inport  Port=3
  1/Lq : Gain  Gain=1/Lq
  Ld/Lq : Gain  Gain=Ld/Lq
  Product : Product  RndMeth=Zero
  R/Lq : Gain  Gain=R/Lq
  Subtract : Sum  Inputs=---+
  d/dt(iq) : Integrator
  flux/Lq : Gain  Gain=Flux/Lq
  iq : Outport
  wires:
  d/dt(iq)/1 -> iq/1, R/Lq/1
  Subtract/1 -> d/dt(iq)/1
  R/Lq/1 -> Subtract/1
  Ld/Lq/1 -> Subtract/2
  flux/Lq/1 -> Subtract/3
  1/Lq/1 -> Subtract/4
  uq/1 -> 1/Lq/1
  we/1 -> Product/2, flux/Lq/1
  id/1 -> Product/1
  Product/1 -> Ld/Lq/1

== system Sixphase_PMSM_VSD_Robj/Six-phae PMSM/Source/is/IClarke ==
  ialpha,ibeta : Inport
  ix,iy : Inport  Port=2
  Fcn1 : Fcn  Expr=u[1]+u[3]
  Fcn2 : Fcn  Expr=-1/2*u[1]+sqrt(3)/2*u[2]-1/2*u[3]-sqrt(3)/2*u[4]
  Fcn3 : Fcn  Expr=-sqrt(3)/2*u[1]+1/2*u[2]+sqrt(3)/2*u[3]+1/2*u[4]
  Fcn4 : Fcn  Expr=-u[2]-u[4]
  Fcn6 : Fcn  Expr=-1/2*u[1]-sqrt(3)/2*u[2]-1/2*u[3]+sqrt(3)/2*u[4]
  Fcn7 : Fcn  Expr=sqrt(3)/2*u[1]+1/2*u[2]-sqrt(3)/2*u[3]+1/2*u[4]
  Mux : Mux  Inputs=6
  Mux2 : Mux  Inputs=2
  iabcuvw : Outport
  wires:
  Mux2/1 -> Fcn1/1, Fcn2/1, Fcn6/1, Fcn7/1, Fcn4/1, Fcn3/1
  Fcn1/1 -> Mux/1
  Fcn2/1 -> Mux/2
  Fcn6/1 -> Mux/3
  Fcn7/1 -> Mux/4
  Fcn3/1 -> Mux/5
  Fcn4/1 -> Mux/6
  Mux/1 -> iabcuvw/1
  ialpha,ibeta/1 -> Mux2/1
  ix,iy/1 -> Mux2/2

== system Sixphase_PMSM_VSD_Robj/Six-phae PMSM/Source/is/IPARK ==
  s,c : Inport
  id,iq : Inport  Port=2
  Demux : Demux  Outputs=2
  Demux1 : Demux  Outputs=2
  Mux : Mux
  Mux1 : Mux  Inputs=2
  ialpha : Fcn  Expr=u[1]*u[4]-u[2]*u[3]
  ibeta : Fcn  Expr=u[1]*u[3]+u[2]*u[4]
  ialpha,ibeta : Outport
  wires:
  Mux/1 -> ibeta/1, ialpha/1
  Demux/2 -> Mux/2
  Demux/1 -> Mux/1
  id,iq/1 -> Demux/1
  Demux1/1 -> Mux/3
  Demux1/2 -> Mux/4
  s,c/1 -> Demux1/1
  ialpha/1 -> Mux1/1
  ibeta/1 -> Mux1/2
  Mux1/1 -> ialpha,ibeta/1

== system Sixphase_PMSM_VSD_Robj/Six-phae PMSM/Source/ix,iy/ix ==
  ux : Inport
  1/Lz : Gain  Gain=1/Lz
  R/Lz : Gain  Gain=R/Lz
  Subtract : Sum  Inputs=-+
  d/dt(ix) : Integrator
  ix : Outport
  wires:
  d/dt(ix)/1 -> ix/1, R/Lz/1
  Subtract/1 -> d/dt(ix)/1
  R/Lz/1 -> Subtract/1
  1/Lz/1 -> Subtract/2
  ux/1 -> 1/Lz/1

== system Sixphase_PMSM_VSD_Robj/Six-phae PMSM/Source/ix,iy/iy ==
  uy : Inport
  1/Lz : Gain  Gain=1/Lz
  R/Lz : Gain  Gain=R/Lz
  Subtract : Sum  Inputs=-+
  d/dt(iy) : Integrator
  iy : Outport
  wires:
  d/dt(iy)/1 -> iy/1, R/Lz/1
  Subtract/1 -> d/dt(iy)/1
  R/Lz/1 -> Subtract/1
  1/Lz/1 -> Subtract/2
  uy/1 -> 1/Lz/1
